simulink model "neural_controller"  (R2018a)
settings: Solver=VariableStepAuto  StartTime=0.0  StopTime=60  RelTol=1e-3
undefined symbols (not defined in the file or in its folder): now
libraries: neural x1
settings Model: Creator=Rafael  LastModifiedBy=Rafael

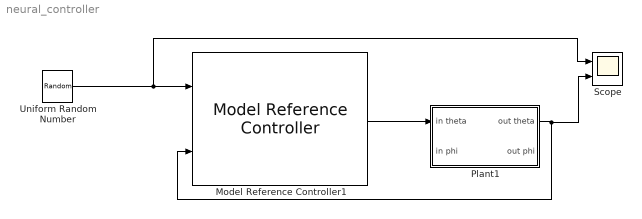
== system neural_controller ==
  Model Reference Controller1 : neural/Control Systems/Model Reference Controller  Nrc=5  Nic=2  Njc=5  IW_y=[2.7797525574294001949 -12.820173475926461393 -13.981707679262305177 4.2193584138540041195 6.7841997576506622991;-1254.7025067598649457 -843.89654927164690434 -495.81506359672863482 -284.72867496725092451 -163.54198143528728338;-41.334584207754815566 30.811730346650168855 37.805143078788731259 30.185445435778056833 22.374865220170875091;-0.7345309189261332028 -0.60642819016053239878 -0.80502114909999833436 -0.50070178389711506028 0.59295189000913106625;-3.4808924875749824857 -0.90092671898587739499 -1.0965284672092032725 0.011497459881772781332 -0.18231773588831112765;-432.66222917664163106 -227.36316606431279297 -114.36443559641537604 -53.799893498107877576 -22.696660534227259376;0.74589190240499014806 0.64149209484767411027 -0.48034700477408642794 -0.66621418220350792083 -0.16778534061393959864;-2.2420769982480432958 0.3332913345628520374 0.52842331519943264162 1.7516232018872983645 1.3965329896310225699;16.853984620111493342 9.4921270743049745988 7.0783381279014250254 23.7566018296309025 35.221165023374759073;-6.5731156477237719926 -2.0452117504388866998 -2.01789149930679379 -0.21269388134621003417 0.060624805971116690895;-7.5096178709088130532 -4.0417814174127109084 -1.9129912617559803323 -0.26932270740031538647 -0.65295770098010941229;-0.71910948112172379254 -1.0486678301021021831 -1.7511908274144232234 -0.96348623657050569413 -1.9245272279152971784;-7.010271811919043472 -2.694371007852240929 -1.5952882588813575016 0.097367777377137851302 -0.53267794088881148529;0.18074166681800185597 0.23212113880736240379 -0.13246566314389612851 0.60424211826773044365 0.34992856274142297712;0.2995090970450615675 0.0093889464109307655543 0.51456528003727808329 -0.24383358870104737681 -0.10501511254798941153;-1.9028340565093306846 -1.2326205634327838112 0.4475299692150307429 -0.36931852543904097885 -0.0059306225454010021159;497.81865507446400443 297.11884833627016178 182.88767581991865541 111.30635254831315706 66.174851237883729027;-70.413895004967258728 -37.587447571235763633 -16.739606165212098432 -4.8657245687443655413 -2.2430000706173900404;-4.9249101723133810182 -2.7989956498710606425 -0.57800508288516061484 -0.88547514692797002489 -0.44659706198612736383;-0.70157245135806867165 -0.072585138745824326345 0.65697368833862845872 -0.018426388691032708628 -0.30145132951083813966;-9.2723503020243409622 -1.5975050636154757289 0.50622460975143868112 -0.66958541861267983908 0.86367125029659785884;-26.252421834723524086 -13.395798871921847706 -5.2833738516521560058 -1.1745625788754483487 0.3422484217291554276;5.3243998225282389569 1.6194387521695154941 0.093962590857886107987 0.87030193665791266699 0.2906140066033007785;39.734464829810526965 19.234165019421094911 8.4238979622807477199 3.6916644503259754551 1.6838331466227631772;-111.33321994030019653 -79.440973183103650967 -54.444395532226501189 -35.627638685992216949 -22.673802930136275791;104.46675570993075155 51.639393925739966562 24.111341471601377862 10.190688881405312927 2.2781990796399438359;-135.63623459162556628 -77.189779137269368903 -43.557338979807369128 -23.390960984943070855 -11.602900186295917351;-54.697036734837929828 -26.023162263189771437 -11.670795072551287674 -3.727160056989372805 -1.6016165168184608447;-74.909739788539752681 -35.524424420194371521 -13.888211123070052011 -3.550494559934797234 -1.8042375460820145872;-727.91957559808361111 -419.04425111322382236 -237.72642034780500353 -130.8052065559331254 -69.62885902740951849;-12.293629140621229467 -7.1249765871062624711 -2.9020634281713957314 -1.4641024099103350231 -1.2774400097517371044;57.206384656072131634 28.632409424246230145 13.447710192552589703 5.6784545118895666249 0.97771025842443548548;18.769129762698529618 10.049100391427748136 3.4131982691145275055 -0.45618971963005544579 -0.34641192247980878705;-2.1630183774026643384 -0.32573394154249885046 -0.5872542867499802588 0.72579321895826853783 -0.36576646244237692729;-154.960233347149682 -79.602655274805769636 -36.852338231181697381 -14.916237673911016515 ...(+1722 chars)]  IW_u=[14.92979651135818564 -336.67376178568247269;-7.8200907827441570319 -4.6397450680758751673;97.498748846208599161 49.871763070666048634;-0.82949001690114210206 1.9576543747238073223;10.674740891318840852 0.96005926312570322168;178.82461719507523412 148.87524996971905011;-0.76928765191739034712 0.072576928473718285706;3.5461408685224728998 -8.9314013438882646767;91.946816884911413581 -68.775181813530466002;13.711055129755765236 2.9160432847738571027;10.481083224250333785 -0.81986038470315314441;48.149567820465414059 -28.532691804431298266;7.5150014669226825603 2.763306532809103544;4.3205732087949453302 -17.187565939330706755;1.356476010028845991 3.9181906678819040657;8.3528102910966897099 0.076273791167682181147;5.6485557250597535628 151.40362029326635707;63.722213342248480217 -32.772746116612943013;16.859217968392488984 3.1304166123251735421;0.28415110892562406297 -1.1677759350832639385;25.750410250756097241 57.137861792832509877;26.003062486537878328 -27.768519881410419714;-15.12334929379173154 -29.784251297237528178;-30.116029864426888452 -17.600628065186214144;-176.02122835615233498 -94.943212198690105197;-80.937858088725235461 -57.610771642088714373;3.3242225369247297984 5.3386687364066087724;49.817114098471002137 5.9689841632851683428;84.935669955401735365 20.488412307490726505;-107.60255065707104905 -1.3347560610817004179;6.8723239080025368963 5.0878260309281886364;-34.495522860746746119 -18.671891859250681733;-18.742287062668804509 21.222462810350634754;7.489786762437179668 0.2559009185689815058;107.1791527810913891 49.420321971175695808;-3.3710428084456518505 -1.6343181259902352931;-17.321859721073366245 2.5702357060889116092;19.40682658638377589 -32.023031458536131311;-18.302076349541863465 12.246085557381972464;-77.485193440865074876 -76.149480136356984872;-17.393344099464719932 -10.654500006465625006;-27.511616994807326364 0.82863810232683188239;-2.1533063274764203676 36.094557870026314106;6.6181960886180242198 -2.1633045661278096361;133.6728801921979084 96.812497268739249989;-56.192326589355779731 -28.220595593846542926;63.508021088789412545 50.654860931926272372;7.3400824800209765186 -3.6264697744140281799;-32.640829745634825088 -34.486984061711993377;0.91666450620755035583 -17.167885645559831431]  IW_r=[0.83364173646733819023 -0.1046121572011874945 -0.24260628261759922819 -0.84109626074278942554 -0.1236714520200177525;-1.1556739861079410314 -0.99940040621488879236 -2.0490647867393296799 -0.73657135202770318561 -0.29939239039665110909;2.1605245050726362699 2.0336498958611395338 1.8673652313620017207 6.267426937190680114 3.6086581942683708668;1.0061530489060692695 0.4383371549670238565 -0.33674701729147965557 -0.57127942113708407579 0.10787138987577225835;0.71893414097580743416 1.5208957389313828568 0.91375761033752755935 -0.13143383571672870302 0.16662211988644118343;6.3732679618577661174 6.4902054207973236544 5.3720167564275476124 6.9473429241534541134 6.6398534450103925408;0.25035568602399504989 -0.081375556842238169764 -0.76326092127138400745 -0.83062841670563369867 -0.6524006820259025119;-0.73386715202551699999 0.070921168721965646697 0.059369050080782588552 -0.68354538284170107687 0.43339001377738783916;-0.71958068281838349911 0.29583921366312293522 -0.76671587479364011752 -0.21389634502408608197 0.50405285842461933221;1.2874075109923124316 1.3405415594410412528 -0.04015343512570269946 0.57634696402872476195 -0.015415975211308968751;1.3264371398029839444 0.67058210606816415211 0.50386543150521656553 0.2734639165497970148 0.69320344898568575509;-1.115412595544851948 0.48369112729160901321 -0.56455390050488440945 0.40372533499148111069 0.56245673661527628706;-0.12150192965176284665 0.34393365319743829378 0.67182880250165155633 0.69627472675943169467 0.039805051437893125554;-0.61411093007690642498 -0.044886331347641382494 -0.27020290492933118909 1.6812578466381835618 0.55293366829275591989;-0.18318723182346757783 -0.65519004770827538042 0.1655111306048113462 -0.82298661265474681858 0.32689693029695421345;1.1580940867490063795 1.283469296232353285 -0.29301013040057244385 0.99454038431059721415 0.85169809232588045145;-2.9639161114322090107 -2.8842237064807774161 -0.42320886405318486334 -1.249270225870027673 1.4463532249251462858;1.6987692364059838734 0.18765121803243159371 -0.21475800666077865531 7.320127281559571486 2.5235078832843491625;1.1629130284888398172 0.58996676604812037237 0.82353902043534121802 0.19475452017947395 0.066100768467551501706;0.1664933096544445601 0.84582936910831729715 -0.04577150629849542629 0.015965329876733869857 -0.64008145448525133325;2.6946796981021425843 3.1123076666737872209 3.7669789656038275005 -1.8247274767823120634 0.49488030110772335268;1.0571727315832597505 -0.8574832874453363063 -0.92372802039788204365 5.6790615398416566251 0.87818938693767789605;-1.0634502722109397954 -1.6728961875475707455 -2.1768099312550996949 0.21214640999576919733 -0.6526915108956695688;-1.47900702949592322 -2.0708425328746722371 -1.1741189872735613431 -1.2461519718850400107 -1.550401646922505261;-6.6027178100426349161 -7.0616731310456932746 -4.9944604292173462312 -6.2338278652062060203 -4.0837510012313629204;-4.2765371391268844903 -3.0703889855698092148 -2.8290367183895437364 -3.6937989357019538339 -2.7902007416437193399;0.11040142739807304317 0.72058045871000042659 0.52966652244860734644 0.48635364910884426592 1.1187625681702297875;2.0494676539386440517 2.3833743047586581909 0.15335351890686116372 3.6742954628106510029 1.0262112769922464572;4.367062678052363367 4.0717653128265700602 2.0054601434079217803 7.1097735905888850283 1.7029480925227828969;-2.6443175299715067084 -2.3453744368994322578 -1.7476045578051526697 -3.4966855018896181306 0.47448518117119203863;0.56291099196167315721 0.769149061860184724 0.12786501576804004676 1.732087054388558256 0.059911467175234260629;-0.97756341788259248915 -0.30078773194880853437 -0.79167450246594506247 -1.4232285875007728571 -1.3021411976851113845;0.87167866415377093237 0.091611426933885839463 -0.68015118772691773863 -4.8467182044528378526 0.46671930176763409825;-0.052977143688391688248 -0.40596691656244898727 0.24713946317093254956 0.90095207260262788473 0.60368341753143495154;2.251747370816775895 2.2402175730790934161 2.9244158934150741302 6.8555568635409613876 ...(+1750 chars)]  B1_c=[0.72463991618480727563;-2.759592692944890846;12.519548631607257505;1.9089699563386890446;2.0448468211080128576;40.433209795542417453;3.5596338941809264611;0.33222810647981765309;-5.506519561882561753;3.9677215455647463216;4.3708768875562267198;-6.1854780508184656895;4.2250606335434213179;-2.7863713567735306498;4.233776485919552357;4.7311376093456889436;-17.468591523153786937;6.2830608267910905695;7.7543758992799665108;-2.9287943061356531693;19.766905714032546371;3.5403965694942738374;-10.488602437961887404;-8.1798542882031455292;-41.364463585272709167;-21.526180645452640761;3.77881159424981794;11.135729143203887404;26.043136102840385604;-20.979097132234720391;0.94915187632103104054;-5.4377183081386455399;4.5099487251977521396;3.5243676269309114346;19.434261121343158862;-2.4868839809967213661;-4.3264436103515935272;5.2489786113310108462;-4.0593591239462609721;-19.965462862741869543;-6.243181344350182016;-10.885481372435057423;8.8284650845780188178;-3.1706729050600808151;31.771457420991421117;-24.129384993680979221;16.228678025663064943;2.8528098503083785253;-5.7556764692291997321;-2.6945599017785388796]  B2_c=1189.8037921672842003  LW_c=[1246.3069886429436792 306.99402007664906478 -389.70289532861096404 -1422.406190287444133 -2036.7379784694107911 -2224.8158868810724016 3273.4667435875862793 575.85342786471812815 -1142.6797460846655667 465.03232647419406476 -1191.8468639829493441 -708.0880007893073298 -3313.5845690637152074 -1636.6235875573740941 -250.15111386828951368 485.72372621804714754 2437.9581908723957895 -198.44038687018291967 -641.05855460423708791 -1498.0306695346835113 1463.2251377398843033 1556.8472489560062968 2165.8318153793825331 1472.6239233537191922 -1373.1247558295949602 -1660.4115484169840329 -710.48757047408753351 440.55428162261802072 202.19191707585878248 -1090.4013110151458932 -991.28115053317083039 1763.1659157857325226 -1654.4175421638194621 -750.94179339327627076 -4264.0574115131312283 -1028.6041837519185265 26.753119028459042994 1576.0072687470837991 3022.1979972905960494 3382.9733621622281134 421.43690258575804819 1408.8488732748232906 -1765.8925506292118826 -631.06346436001945222 1616.8608601284606721 -213.39782329113367609 -1657.0411269378121233 1567.9986737813674154 1290.0458259423080563 -611.85214078878391319]  retraining_c=30  max_i_int=2  min_i_int=0.1  max_r_int=2  min_r_int=0.1  Ts=0.05  S1=10  Ni=2  Nj=2  sim_file=model  trainfun=trainlm  Use_validation=1  Use_Testing=1  Use_Inc_training=0  Use_previous_weights=1  max_i=90  min_i=-90  max_r=90  min_r=-90  sam_training=10000  sam_training_c=1000  epochs=300  epochs_c=10  minp=-89.958408264104988916  maxp=89.96266160005529855  mint=-173.15895607331853512  maxt=89.96266160005529855  Normalize=0  IW=[-0.00011351218881326583757 -0.00010663863417005723831;-0.00090741291856376543427 -9.9483434124820370871e-05;-0.33656743355117435534 -0.24885275928285624514;0.19287062337298305215 2.8661482362474330898;-0.00035223797321260185171 -0.00022316091209240702486;-1.1142393362588496331 0.66067083391645087254;0.020263255378609325297 -0.0087783956444444331824;-0.00062066779219760242429 -0.00020705274741932092877;1.1834374334841133436 -0.97826630923860391498;-0.39745703452032515868 0.73907781345790490857]  LW1_2=[0.0044104871769779013455 -0.0019329838124019925634;0.027467355936674240496 -0.014568351807862778627;-14.164210331911815999 12.505416146402570376;11.765113345087389263 3.8325731682201338302;0.012544030961649844241 -0.0059037186710604455664;-17.549810752044606943 1.684315659887231309;-0.28147980493358676357 0.074746033506931028323;0.020175664099462298912 -0.010178280650944686661;11.829384368111934833 -9.414795297319033196;8.7140413919767620854 -10.91554483318055091]  LW2_1=[713.34757072445165704 -7.6373731294387523505 -0.00087538545067267355907 2.3483443235329866546e-05 -109.02556137710878659 -0.0011837774183791403664 -0.0043720357680233608647 36.864475110984031403 0.001583848898063267745 0.0019634719187187083672]  B1=[0.00020213159451297393193;0.0039134905831659117653;-85.233866420542071296;15.128428127755190857;0.00088788344618001362706;6.5797192805094395496;-1.2853036731130678127;0.0021357107732533804623;-72.041414458734394088;-16.167015752450716093]  B2=-0.096782640257189217481  S1c=50  Limit_output=1  min_output=-90  max_output=90  Ref_file=model
      settings: SourceProductName=Neural Network Toolbox  SourceProductBaseCode=NN
  Plant1 : Subsystem
  Scope : Scope  NumInputPorts=2
  Uniform Random Number : UniformRandomNumber  Minimum=-90  Maximum=90  Seed=round(now)  SampleTime=10
  wires:
  Plant1/1(out theta) -> Model Reference Controller1/2, Scope/2
  Uniform Random Number/1 -> Model Reference Controller1/1, Scope/1
  Model Reference Controller1/1 -> Plant1/1(in theta)

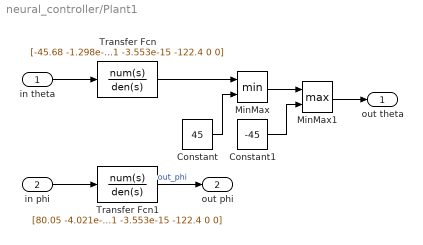
== system neural_controller/Plant1 ==
  in theta : Inport
  in phi : Inport  Port=2
  Constant : Constant  Value=45
  Constant1 : Constant  Value=-45
  MinMax : MinMax  Inputs=2
  MinMax1 : MinMax  Function=max  Inputs=2
  Transfer Fcn : TransferFcn  Numerator=[-45.68 -1.298e-11 7.179e-13]  Denominator=[1 -3.553e-15 -122.4 0 0]
  Transfer Fcn1 : TransferFcn  Numerator=[80.05 -4.021e-12 61140]  Denominator=[1 -3.553e-15 -122.4 0 0]
  out theta : Outport
  out phi : Outport  Port=2
  wires:
  Transfer Fcn1/1 -> out phi/1  "out_phi"
  in theta/1 -> Transfer Fcn/1
  in phi/1 -> Transfer Fcn1/1
  Constant1/1 -> MinMax1/2
  Constant/1 -> MinMax/2
  Transfer Fcn/1 -> MinMax/1
  MinMax/1 -> MinMax1/1
  MinMax1/1 -> out theta/1
